simulink model "bang_bang_hist_DI_PD"  (R2020a)
settings: Solver=ode45  StartTime=0.0  StopTime=20  MaxStep=1e-5  RelTol=1e-3  EnableMultiTasking=on
values from neighbouring files (symbols this model uses):
  a = 3    [Tito_Ricardo_Clemente_Tarea_3.m]
  K = 10    [Ray.m]    (also in Tito_Riacrdo_Clemente_Tarea_3_PID.m = 5; Tito_Ricardo_Clemente_Tarea_3.m = 5)
  Kc = 0.53046    [Tito_Ricardo_Clemente_Tarea_3.m]
  lineal = 0    [Tito_Ricardo_Clemente_Tarea_3.m]
  M = Kc    (= 0.53046)    [Tito_Ricardo_Clemente_Tarea_3.m]
  p1 = -3    [Ray.m]    (also in Tito_Riacrdo_Clemente_Tarea_3_PID.m = -1; Tito_Ricardo_Clemente_Tarea_3.m = -1)
  p2 = 4    [Ray.m]    (also in Tito_Riacrdo_Clemente_Tarea_3_PID.m = 2; Tito_Ricardo_Clemente_Tarea_3.m = 2)
  T = 0.23    [Tito_Riacrdo_Clemente_Tarea_3_PID.m]    (also in Tito_Ricardo_Clemente_Tarea_3.m = 0.026523)
settings Model: Creator=Usuario  LastModifiedBy=Usuario
settings DataIOCC: SaveFormat=Array  SignalLoggingSaveFormat=ModelDataLogs  ReturnWorkspaceOutputs=off
settings OptimizationCC: BlockReduction=off  BooleanDataType=off  InitFltsAndDblsToZero=on  LifeSpan=inf
settings DebuggingCC: SaveWithParameterizedLinksMsg=none  UnderspecifiedInitializationDetection=Classic  MergeDetectMultiDrivingBlocksExec=none  SignalResolutionControl=TryResolveAllWithWarning  MultiTaskDSMMsg=warning  MultiTaskCondExecSysMsg=none  FcnCallInpInsideContextMsg=warning  SFUnexpectedBacktrackingDiag=warning  SFNoUnconditionalDefaultTransitionDiag=warning  SFExecutionAtInitializationDiag=none  ArithmeticOperatorsInVariantConditions=warning
settings HardwareCC: ProdBitPerPointer=32  ProdBitPerSizeT=32  ProdBitPerPtrDiffT=32  ProdLargestAtomicFloat=None  ProdIntDivRoundTo=Undefined  ProdEndianess=Unspecified  ProdWordSize=32  ProdHWDeviceType=32-bit Generic  TargetUnknown=on
settings ModelReferenceCC: PropagateSignalLabelsOutOfModel=off
settings SFSimCC: SimUseLocalCustomCode=off  CustomCodeUndefinedFunction=UseInterfaceOnly
settings RTWCC: Description=Generic Real-Time Target  RTWUseLocalCustomCode=off
settings CodeAppCC: StateflowObjectComments=on
settings GRTTargetCC: TargetFcnLib=ansi_tfl_tmw.mat  TargetLangStandard=C89/C90 (ANSI)  CombineOutputUpdateFcns=off  GRTInterface=on
settings ConfigComp: CovMetricSettings=dw  CovHtmlReporting=on  CovSaveCumulativeToWorkspaceVar=on  CovSaveSingleToWorkspaceVar=on  CovExternalEMLEnable=off  CovSFcnEnable=off

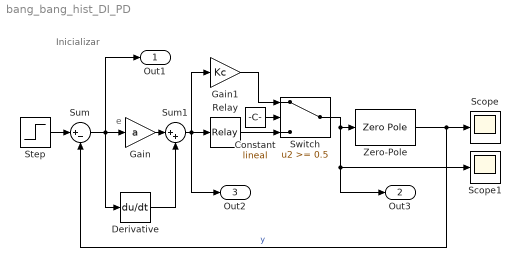
== system bang_bang_hist_DI_PD ==
  note: Inicializar
  note: e
  Constant : Constant  Value=lineal
  Derivative : Derivative
  Gain : Gain  Gain=a
  Gain1 : Gain  Gain=Kc
  Relay : Relay  OnSwitchValue=T  OffSwitchValue=-T  OnOutputValue=M  OffOutputValue=-M
  Scope : Scope
  Scope1 : Scope
  Step : Step  Time=0  SampleTime=0
  Sum : Sum  Inputs=|+-  InputSameDT=on  SaturateOnIntegerOverflow=on  OutDataTypeStr=Inherit: Same as first input
  Sum1 : Sum  Inputs=|++
  Switch : Switch  Threshold=0.5
  Zero-Pole : ZeroPole  Zeros=[]  Poles=[p2 p1]  Gain=[K]
  Out1 : Outport
  Out3 : Outport  Port=2
  Out2 : Outport  Port=3
  wires:
  Zero-Pole/1 -> Sum/2, Scope/1  "y"
  Step/1 -> Sum/1
  Derivative/1 -> Sum1/2
  Sum/1 -> Gain/1, Out1/1, Derivative/1
  Gain/1 -> Sum1/1
  Relay/1 -> Switch/3
  Switch/1 -> Out3/1, Scope1/1, Zero-Pole/1
  Sum1/1 -> Gain1/1, Out2/1, Relay/1
  Gain1/1 -> Switch/1
  Constant/1 -> Switch/2
